simulink model "StepByStep_CR"  (R2014b)
settings: Solver=ode45  StartTime=0.0  StopTime=150  RelTol=1e-3
values from neighbouring files (symbols this model uses):
  B1 = round(B1,6)    [liniarizare_crazyflie.m]
undefined symbols (not defined in the file or in its folder): A1, C1, D1
settings Model: Creator=uidd7441  LastModifiedBy=uidd7441
settings DataIOCC: SignalLogging=off

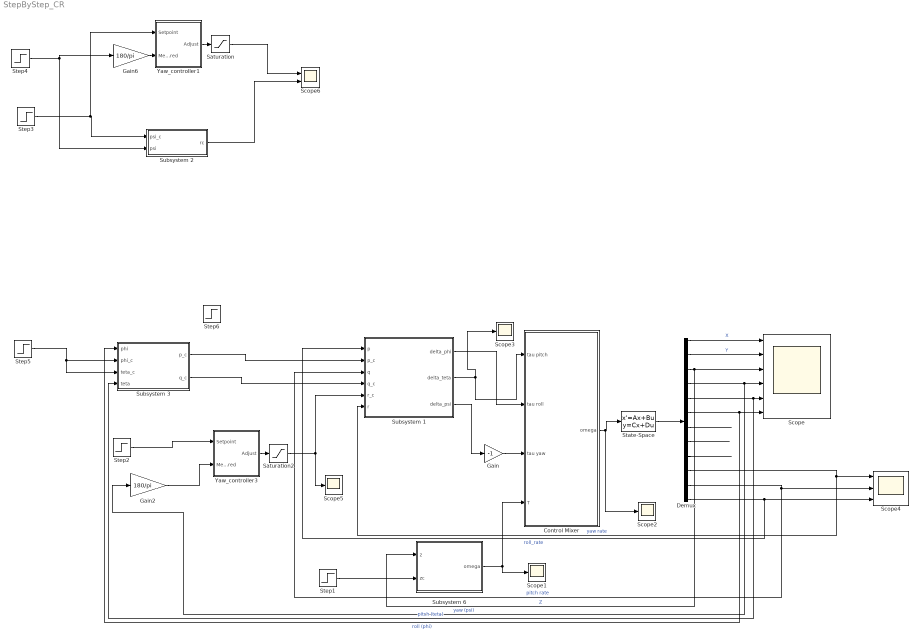
== system StepByStep_CR ==
  Control Mixer : Subsystem  AncestorBlock=roblocks/Dynamics/Control Mixer 4
      mask help: Quadrotor control mixer
      mask Help:
      | Determine rotor speeds based on desired torques and thrust.
      | 
      | <b>Inputs::</b>
      | 
      | tau pitch (1x1)  desired pitching torque [Nm]
      | tau roll (1x1)   desired rolling torque [Nm]
      | tau yaw (1x1)    desired yawing torque [Nm]
      | T (1x1)          desired thrust [N]
      | 
      | <b>Outputs::</b>
      | 
      | w1 (1x1) angular velocity of rotor 1 [rad]
      | w2 (1x1) angular velocity of rotor 2 [rad]
      | w3 (1x1) angular velocity of rotor 3 [rad]
      | w4 (1x1) angular velocity of rotor 4 [rad]
      | 
      | <b>Notes::</b>
      | 
      | - Assumes the rotor labelling convention of RVC Fig 4.16.
      | - The quadrotor is underactuated and has only 4 inputs.
  Demux : Demux  Outputs=12
  Gain : Gain  Gain=-1
  Gain2 : Gain  Gain=180/pi
  Gain6 : Gain  Gain=180/pi
  Saturation : Saturate  UpperLimit=200  LowerLimit=-200
  Saturation2 : Saturate  UpperLimit=200  LowerLimit=-200
  Scope : Scope  NumInputPorts=6
      settings: YMin=-5~-5~-5~-5~-5~-5  YMax=5~5~5~5~5~5
  Scope{1..3,5} (4 alike) : Scope
      Scope2 settings: SaveName=ScopeData2
      Scope3 settings: TimeRange=150  YMin=0  YMax=70  SaveName=ScopeData3
      Scope5 settings: TimeRange=150  YMin=0  YMax=70  SaveName=ScopeData4
  Scope4 : Scope  NumInputPorts=3
      settings: YMin=-5~-5~-5  YMax=5~5~5  SaveName=ScopeData5
  Scope6 : Scope  NumInputPorts=2
      settings: YMin=-5~-5  YMax=5~5  SaveName=ScopeData11
  State-Space : StateSpace  A=A1  B=B1  C=C1  D=D1  X0=[0 0 0 0 0 0 0 0 0 0 0 0]'
  Step{1,4..6} (4 alike) : Step  Time=0  SampleTime=0
  Step2 : Step  Time=0  After=0  SampleTime=0
  Step3 : Step  Time=0  After=2  SampleTime=0
  Subsystem 1 : Subsystem
  Subsystem 2 : Subsystem
  Subsystem 3 : Subsystem
  Subsystem 6 : Subsystem
  Yaw_controller1 : Subsystem
  Yaw_controller3 : Subsystem
  wires:
  State-Space/1 -> Demux/1
  Demux/2 -> Scope/2  "Y"
  Demux/1 -> Scope/1  "X"
  Demux/3 -> Subsystem 6/1(z), Scope/3  "Z"
  Demux/4 -> Gain2/1, Scope/4  "yaw (psi)"
  Demux/5 -> Subsystem 3/4(teta), Scope/5  "pitch (teta)"
  Demux/6 -> Subsystem 3/1("phi "), Scope/6  "roll (phi)"
  Control Mixer/1(omega) -> Scope2/1, State-Space/1
  Subsystem 6/1(omega) -> Control Mixer/4(T), Scope1/1
  Step1/1 -> Subsystem 6/2(zc)
  Subsystem 1/2(delta_teta) -> Control Mixer/1(tau pitch), Scope3/1
  Demux/12 -> Subsystem 1/1(p), Scope4/3  "roll_rate"
  Demux/11 -> Scope4/2, Subsystem 1/3(q)  "pitch rate"
  Subsystem 1/3(delta_psi) -> Gain/1
  Demux/10 -> Scope4/1, Subsystem 1/6(r)  "yaw rate"
  Gain/1 -> Control Mixer/3(tau yaw)
  Step2/1 -> Yaw_controller3/1(Setpoint)
  Yaw_controller1/1(Adjust) -> Saturation/1
  Gain6/1 -> Yaw_controller1/2(Measured)
  Saturation/1 -> Scope6/1
  Subsystem 2/1(rc) -> Scope6/2
  Yaw_controller3/1(Adjust) -> Saturation2/1
  Gain2/1 -> Yaw_controller3/2(Measured)
  Step3/1 -> Yaw_controller1/1(Setpoint), Subsystem 2/1(psi_c)
  Step4/1 -> Gain6/1, Subsystem 2/2(psi)
  Saturation2/1 -> Scope5/1, Subsystem 1/5(r_c)
  Subsystem 1/1(delta_phi) -> Control Mixer/2(tau roll)
  Step5/1 -> Subsystem 3/3(teta_c), Subsystem 3/2(phi_c)
  Demux/7 -> ?
  Demux/8 -> ?
  Demux/9 -> ?
  Subsystem 3/1(p_c) -> Subsystem 1/2(p_c)
  Subsystem 3/2(q_c) -> Subsystem 1/4(q_c)

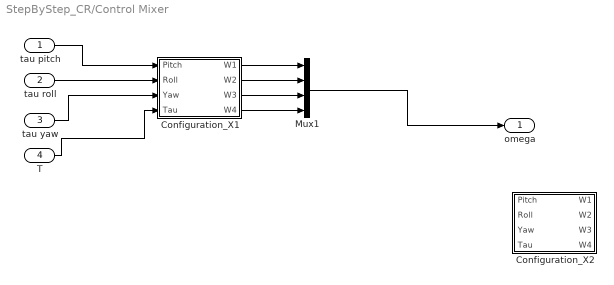
== system StepByStep_CR/Control Mixer ==
  tau pitch : Inport
  tau roll : Inport  Port=2
  tau yaw : Inport  Port=3
  T : Inport  Port=4
  Configuration_X1 : Subsystem
  Configuration_X2 : Subsystem
  Mux1 : Mux
  omega : Outport
  wires:
  Configuration_X1/1(W1) -> Mux1/1
  Configuration_X1/2(W2) -> Mux1/2
  Configuration_X1/3(W3) -> Mux1/3
  Configuration_X1/4(W4) -> Mux1/4
  tau pitch/1 -> Configuration_X1/1(Pitch)
  tau roll/1 -> Configuration_X1/2(Roll)
  tau yaw/1 -> Configuration_X1/3(Yaw)
  T/1 -> Configuration_X1/4(Tau)
  Mux1/1 -> omega/1

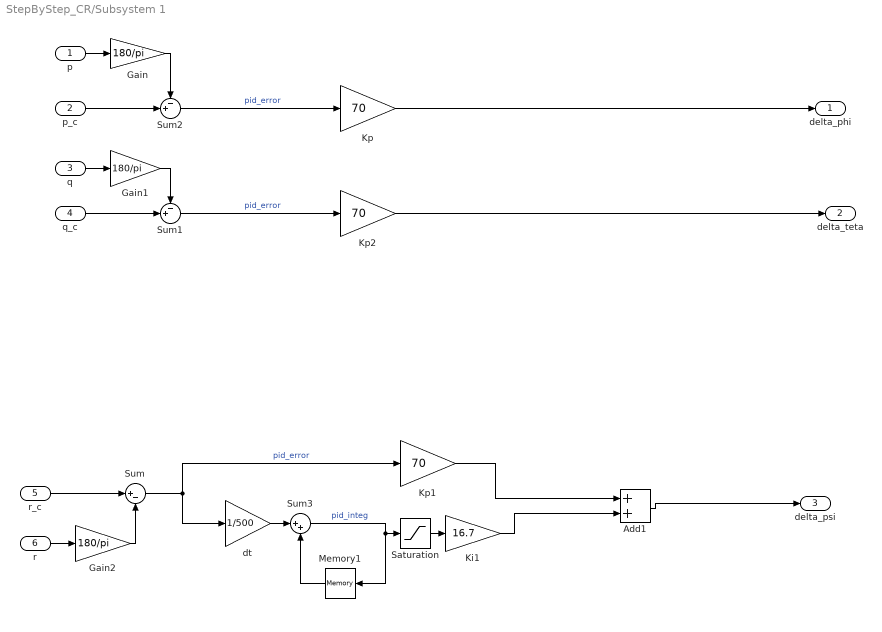
== system StepByStep_CR/Subsystem 1 ==
  p : Inport
  p_c : Inport  Port=2
  q : Inport  Port=3
  q_c : Inport  Port=4
  r_c : Inport  Port=5
  r : Inport  Port=6
  Add1 : Sum
  Gain : Gain  Gain=180/pi
  Gain1 : Gain  Gain=180/pi
  Gain2 : Gain  Gain=180/pi
  Ki1 : Gain  Gain=16.7  OutMin=[-200]  OutMax=[200]
  Kp : Gain  Gain=70  OutMin=[-200]  OutMax=[200]
  Kp1 : Gain  Gain=70  OutMin=[-200]  OutMax=[200]
  Kp2 : Gain  Gain=70  OutMin=[-200]  OutMax=[200]
  Memory1 : Memory
  Saturation : Saturate  UpperLimit=166.7  LowerLimit=-166.7
  Sum : Sum  Inputs=|+-
  Sum1 : Sum  Inputs=-+|
  Sum2 : Sum  Inputs=-+|
  Sum3 : Sum  Inputs=|++
  dt : Gain  Gain=1/500  OutMin=[-200]  OutMax=[200]
  delta_phi : Outport
  delta_teta : Outport  Port=2
  delta_psi : Outport  Port=3
  wires:
  Gain2/1 -> Sum/2
  Gain1/1 -> Sum1/1
  Gain/1 -> Sum2/1
  Saturation/1 -> Ki1/1
  Memory1/1 -> Sum3/2
  Sum3/1 -> Memory1/1, Saturation/1  "pid_integ"
  dt/1 -> Sum3/1
  Ki1/1 -> Add1/2
  Kp1/1 -> Add1/1
  Sum2/1 -> Kp/1  "pid_error"
  Add1/1 -> delta_psi/1
  Kp/1 -> delta_phi/1
  r/1 -> Gain2/1
  r_c/1 -> Sum/1
  p/1 -> Gain/1
  p_c/1 -> Sum2/2
  q_c/1 -> Sum1/2
  q/1 -> Gain1/1
  Sum1/1 -> Kp2/1  "pid_error"
  Kp2/1 -> delta_teta/1
  Sum/1 -> dt/1, Kp1/1  "pid_error"

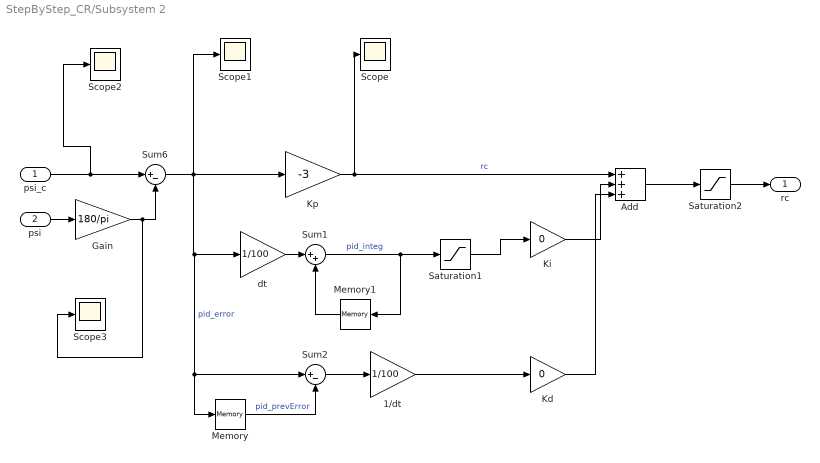
== system StepByStep_CR/Subsystem 2 ==
  psi_c : Inport
  psi : Inport  Port=2
  1/dt : Gain  Gain=1/100  OutMin=[-200]  OutMax=[200]
  Add : Sum  Inputs=+++
  Gain : Gain  Gain=180/pi
  Kd : Gain  Gain=0  OutMin=[-200]  OutMax=[200]
  Ki : Gain  Gain=0  OutMin=[-200]  OutMax=[200]
  Kp : Gain  Gain=-3  OutMin=[-200]  OutMax=[200]
  Memory : Memory
  Memory1 : Memory
  Saturation1 : Saturate  UpperLimit=166.7  LowerLimit=-166.7
  Saturation2 : Saturate  UpperLimit=200  LowerLimit=-200
  Scope{,1..3} (4 alike) : Scope
      Scope settings: SaveName=ScopeData6
      Scope1 settings: SaveName=ScopeData7
      Scope2 settings: SaveName=ScopeData8
      Scope3 settings: SaveName=ScopeData9
  Sum1 : Sum  Inputs=|++
  Sum2 : Sum  Inputs=|+-
  Sum6 : Sum  Inputs=|+-
  dt : Gain  Gain=1/100  OutMin=[-200]  OutMax=[200]
  rc : Outport
  wires:
  Saturation2/1 -> rc/1
  Add/1 -> Saturation2/1
  Memory/1 -> Sum2/2  "pid_prevError"
  Ki/1 -> Add/2
  Kd/1 -> Add/3
  dt/1 -> Sum1/1
  Sum2/1 -> 1/dt/1
  1/dt/1 -> Kd/1
  Sum6/1 -> Kp/1, Scope1/1, dt/1, Memory/1, Sum2/1  "pid_error"
  Sum1/1 -> Memory1/1, Saturation1/1  "pid_integ"
  Memory1/1 -> Sum1/2
  Saturation1/1 -> Ki/1
  Gain/1 -> Sum6/2, Scope3/1
  psi/1 -> Gain/1
  psi_c/1 -> Sum6/1, Scope2/1
  Kp/1 -> Scope/1, Add/1  "rc"

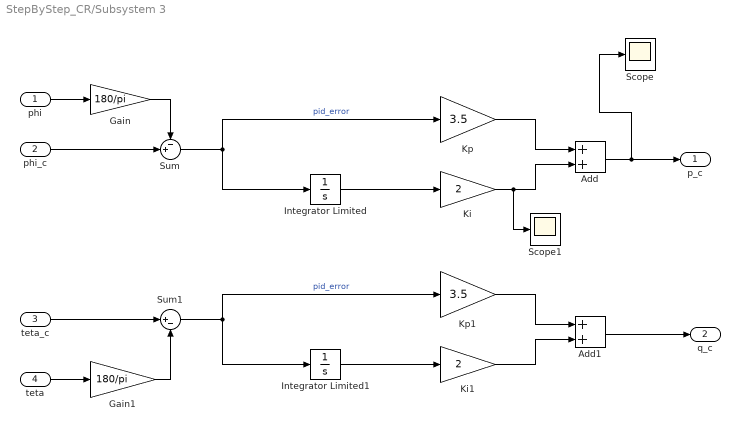
== system StepByStep_CR/Subsystem 3 ==
  "phi " : Inport
  phi_c : Inport  Port=2
  teta_c : Inport  Port=3
  teta : Inport  Port=4
  Add : Sum
  Add1 : Sum
  Gain : Gain  Gain=180/pi
  Gain1 : Gain  Gain=180/pi
  Integrator Limited : Integrator  LimitOutput=on  UpperSaturationLimit=20  LowerSaturationLimit=-20
  Integrator Limited1 : Integrator  LimitOutput=on  UpperSaturationLimit=20  LowerSaturationLimit=-20
  Ki : Gain  Gain=2  OutMin=[-200]  OutMax=[200]
  Ki1 : Gain  Gain=2  OutMin=[-200]  OutMax=[200]
  Kp : Gain  Gain=3.5  OutMin=[-200]  OutMax=[200]
  Kp1 : Gain  Gain=3.5  OutMin=[-200]  OutMax=[200]
  Scope : Scope
      settings: SaveName=ScopeData7
  Scope1 : Scope
      settings: SaveName=ScopeData8
  Sum : Sum  Inputs=-+|
  Sum1 : Sum  Inputs=|+-
  p_c : Outport
  q_c : Outport  Port=2
  wires:
  "phi "/1 -> Gain/1
  phi_c/1 -> Sum/2
  teta_c/1 -> Sum1/1
  teta/1 -> Gain1/1
  Add/1 -> Scope/1, p_c/1
  Add1/1 -> q_c/1
  Sum/1 -> Integrator Limited/1, Kp/1  "pid_error"
  Integrator Limited/1 -> Ki/1
  Kp/1 -> Add/1
  Sum1/1 -> Integrator Limited1/1, Kp1/1  "pid_error"
  Integrator Limited1/1 -> Ki1/1
  Kp1/1 -> Add1/1
  Ki1/1 -> Add1/2
  Gain/1 -> Sum/1
  Gain1/1 -> Sum1/2
  Ki/1 -> Scope1/1, Add/2

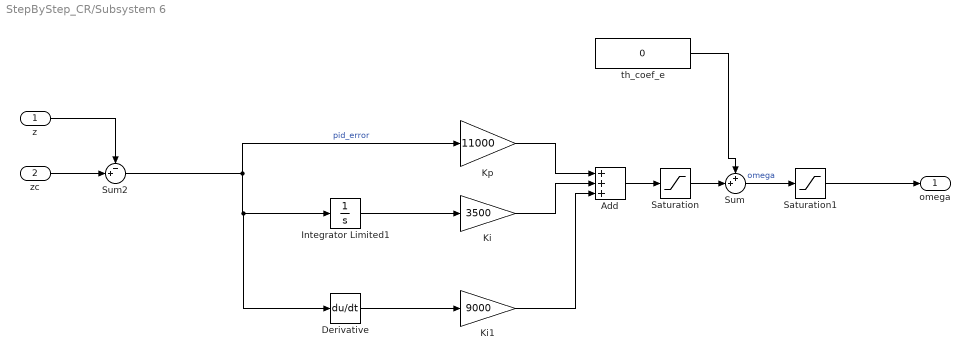
== system StepByStep_CR/Subsystem 6 ==
  z : Inport
  zc : Inport  Port=2
  Add : Sum  Inputs=+++
  Derivative : Derivative
  Integrator Limited1 : Integrator  LimitOutput=on  UpperSaturationLimit=1000  LowerSaturationLimit=-1000
  Ki : Gain  Gain=3500  OutMin=[-200]  OutMax=[200]
  Ki1 : Gain  Gain=9000  OutMin=[-200]  OutMax=[200]
  Kp : Gain  Gain=11000  OutMin=[-200]  OutMax=[200]
  Saturation : Saturate  UpperLimit=15000  LowerLimit=-20000
  Saturation1 : Saturate  UpperLimit=60000  LowerLimit=-20000
  Sum : Sum  Inputs=++|
  Sum2 : Sum  Inputs=-+|
  "th_coef_e " : Constant  Value=0
  omega : Outport
  wires:
  "th_coef_e "/1 -> Sum/1
  Sum/1 -> Saturation1/1  "omega"
  zc/1 -> Sum2/2
  z/1 -> Sum2/1
  Sum2/1 -> Derivative/1, Integrator Limited1/1, Kp/1  "pid_error"
  Integrator Limited1/1 -> Ki/1
  Kp/1 -> Add/1
  Ki/1 -> Add/2
  Ki1/1 -> Add/3
  Derivative/1 -> Ki1/1
  Add/1 -> Saturation/1
  Saturation/1 -> Sum/2
  Saturation1/1 -> omega/1

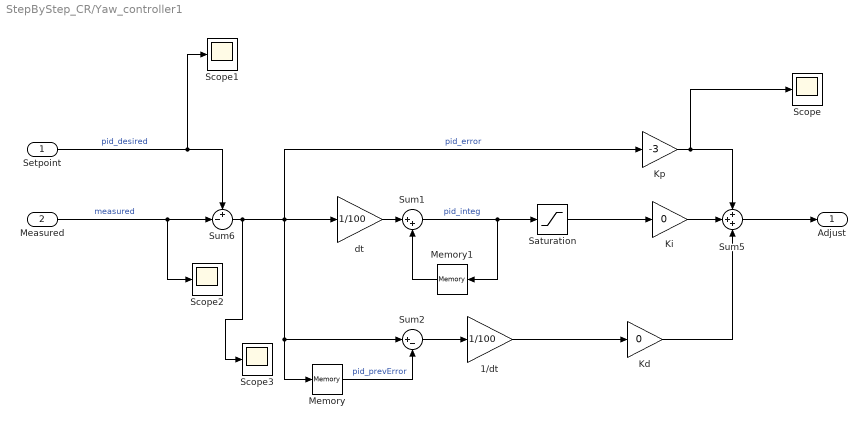
== system StepByStep_CR/Yaw_controller1 ==
  Setpoint : Inport
  Measured : Inport  Port=2
  1/dt : Gain  Gain=1/100  OutMin=[-200]  OutMax=[200]
  Kd : Gain  Gain=0  OutMin=[-200]  OutMax=[200]
  Ki : Gain  Gain=0  OutMin=[-200]  OutMax=[200]
  Kp : Gain  Gain=-3  OutMin=[-200]  OutMax=[200]
  Memory : Memory
  Memory1 : Memory
  Saturation : Saturate  UpperLimit=166.7  LowerLimit=-166.7
  Scope{,1..3} (4 alike) : Scope
      Scope settings: SaveName=ScopeData7
      Scope1 settings: SaveName=ScopeData8
      Scope2 settings: SaveName=ScopeData9
      Scope3 settings: SaveName=ScopeData10
  Sum1 : Sum  Inputs=|++
  Sum2 : Sum  Inputs=|+-
  Sum5 : Sum  Inputs=+++
  Sum6 : Sum  Inputs=+-|
  dt : Gain  Gain=1/100  OutMin=[-200]  OutMax=[200]
  Adjust : Outport
  wires:
  Measured/1 -> Sum6/2, Scope2/1  "measured"
  Setpoint/1 -> Sum6/1, Scope1/1  "pid_desired"
  Memory/1 -> Sum2/2  "pid_prevError"
  Ki/1 -> Sum5/2
  Sum5/1 -> Adjust/1
  Kp/1 -> Sum5/1, Scope/1
  Kd/1 -> Sum5/3
  dt/1 -> Sum1/1
  Sum2/1 -> 1/dt/1
  1/dt/1 -> Kd/1
  Sum6/1 -> Sum2/1, Memory/1, dt/1, Kp/1, Scope3/1  "pid_error"
  Sum1/1 -> Memory1/1, Saturation/1  "pid_integ"
  Memory1/1 -> Sum1/2
  Saturation/1 -> Ki/1

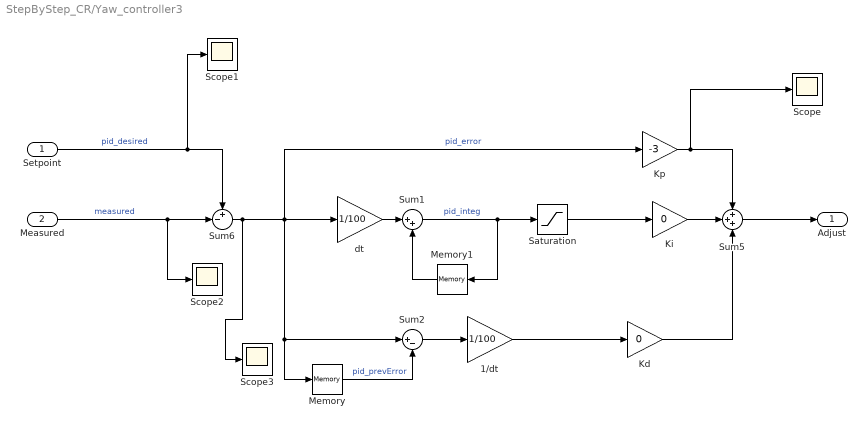
== system StepByStep_CR/Yaw_controller3 ==
  Setpoint : Inport
  Measured : Inport  Port=2
  1/dt : Gain  Gain=1/100  OutMin=[-200]  OutMax=[200]
  Kd : Gain  Gain=0  OutMin=[-200]  OutMax=[200]
  Ki : Gain  Gain=0  OutMin=[-200]  OutMax=[200]
  Kp : Gain  Gain=-3  OutMin=[-200]  OutMax=[200]
  Memory : Memory
  Memory1 : Memory
  Saturation : Saturate  UpperLimit=166.7  LowerLimit=-166.7
  Scope{,1..3} (4 alike) : Scope
      Scope settings: SaveName=ScopeData7
      Scope1 settings: SaveName=ScopeData8
      Scope2 settings: SaveName=ScopeData9
      Scope3 settings: SaveName=ScopeData10
  Sum1 : Sum  Inputs=|++
  Sum2 : Sum  Inputs=|+-
  Sum5 : Sum  Inputs=+++
  Sum6 : Sum  Inputs=+-|
  dt : Gain  Gain=1/100  OutMin=[-200]  OutMax=[200]
  Adjust : Outport
  wires:
  Measured/1 -> Sum6/2, Scope2/1  "measured"
  Setpoint/1 -> Sum6/1, Scope1/1  "pid_desired"
  Memory/1 -> Sum2/2  "pid_prevError"
  Ki/1 -> Sum5/2
  Sum5/1 -> Adjust/1
  Kp/1 -> Sum5/1, Scope/1
  Kd/1 -> Sum5/3
  dt/1 -> Sum1/1
  Sum2/1 -> 1/dt/1
  1/dt/1 -> Kd/1
  Sum6/1 -> Sum2/1, Memory/1, dt/1, Kp/1, Scope3/1  "pid_error"
  Sum1/1 -> Memory1/1, Saturation/1  "pid_integ"
  Memory1/1 -> Sum1/2
  Saturation/1 -> Ki/1

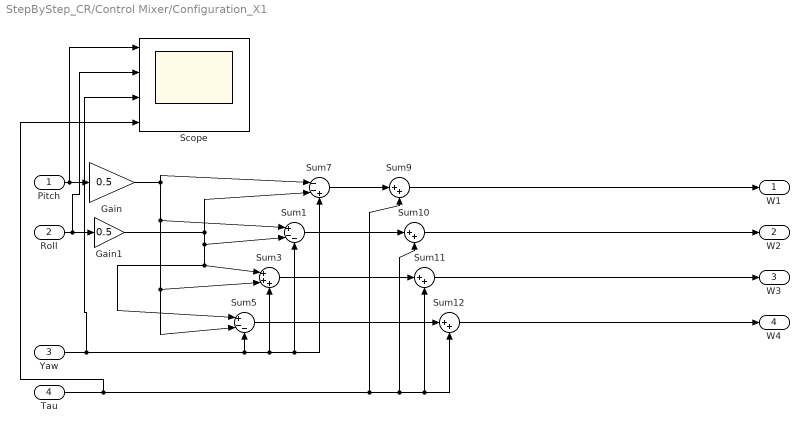
== system StepByStep_CR/Control Mixer/Configuration_X1 ==
  Pitch : Inport
  Roll : Inport  Port=2
  Yaw : Inport  Port=3
  Tau : Inport  Port=4
  Gain : Gain  Gain=0.5
  Gain1 : Gain  Gain=0.5
  Scope : Scope  NumInputPorts=4
      settings: YMin=-5~-5~-5~-5  YMax=5~5~5~5
  Sum1 : Sum  Inputs=|+--  SaturateOnIntegerOverflow=on  InputSameDT=on  OutDataTypeStr=Inherit: Same as first input
  Sum{9..12} (4 alike) : Sum  Inputs=|++  SaturateOnIntegerOverflow=on  InputSameDT=on  OutDataTypeStr=Inherit: Same as first input
  Sum3 : Sum  Inputs=|+++  SaturateOnIntegerOverflow=on  InputSameDT=on  OutDataTypeStr=Inherit: Same as first input
  Sum5 : Sum  Inputs=|+--  SaturateOnIntegerOverflow=on  InputSameDT=on  OutDataTypeStr=Inherit: Same as first input
  Sum7 : Sum  Inputs=|--+  SaturateOnIntegerOverflow=on  InputSameDT=on  OutDataTypeStr=Inherit: Same as first input
  W1 : Outport
  W2 : Outport  Port=2
  W3 : Outport  Port=3
  W4 : Outport  Port=4
  wires:
  Sum3/1 -> Sum11/1
  Yaw/1 -> Sum5/3, Sum3/3, Sum7/3, Sum1/3, Scope/3
  Tau/1 -> Sum11/2, Sum12/2, Sum10/2, Sum9/2, Scope/4
  Sum5/1 -> Sum12/1
  Sum7/1 -> Sum9/1
  Sum1/1 -> Sum10/1
  Roll/1 -> Gain1/1, Scope/2
  Pitch/1 -> Gain/1, Scope/1
  Gain/1 -> Sum7/1, Sum1/1, Sum5/2, Sum3/2
  Gain1/1 -> Sum7/2, Sum1/2, Sum5/1, Sum3/1
  Sum9/1 -> W1/1
  Sum10/1 -> W2/1
  Sum11/1 -> W3/1
  Sum12/1 -> W4/1

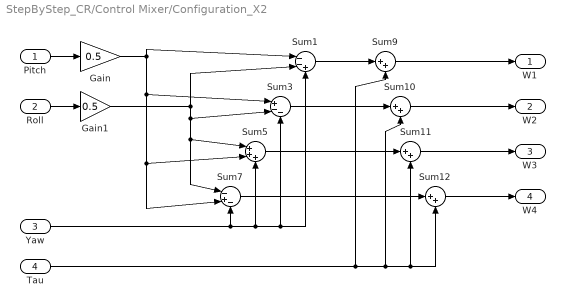
== system StepByStep_CR/Control Mixer/Configuration_X2 ==
  Pitch : Inport
  Roll : Inport  Port=2
  Yaw : Inport  Port=3
  Tau : Inport  Port=4
  Gain : Gain  Gain=0.5
  Gain1 : Gain  Gain=0.5
  Sum1 : Sum  Inputs=|--+  SaturateOnIntegerOverflow=on  InputSameDT=on  OutDataTypeStr=Inherit: Same as first input
  Sum{9..12} (4 alike) : Sum  Inputs=|++  SaturateOnIntegerOverflow=on  InputSameDT=on  OutDataTypeStr=Inherit: Same as first input
  Sum3 : Sum  Inputs=|+--  SaturateOnIntegerOverflow=on  InputSameDT=on  OutDataTypeStr=Inherit: Same as first input
  Sum5 : Sum  Inputs=|+++  SaturateOnIntegerOverflow=on  InputSameDT=on  OutDataTypeStr=Inherit: Same as first input
  Sum7 : Sum  Inputs=|-+-  SaturateOnIntegerOverflow=on  InputSameDT=on  OutDataTypeStr=Inherit: Same as first input
  W1 : Outport
  W2 : Outport  Port=2
  W3 : Outport  Port=3
  W4 : Outport  Port=4
  wires:
  Sum12/1 -> W4/1
  Sum11/1 -> W3/1
  Sum10/1 -> W2/1
  Sum9/1 -> W1/1
  Gain1/1 -> Sum7/1, Sum5/1, Sum3/2, Sum1/2
  Gain/1 -> Sum1/1, Sum5/2, Sum7/2, Sum3/1
  Pitch/1 -> Gain/1
  Roll/1 -> Gain1/1
  Sum3/1 -> Sum10/1
  Sum1/1 -> Sum9/1
  Sum7/1 -> Sum12/1
  Tau/1 -> Sum9/2, Sum10/2, Sum12/2, Sum11/2
  Yaw/1 -> Sum3/3, Sum1/3, Sum5/3, Sum7/3
  Sum5/1 -> Sum11/1
